simulink model "example1Simulink"  (R2023b)
settings: Solver=VariableStepAuto  StartTime=0.0  StopTime=Tsim  RelTol=1e-3
values from neighbouring files (symbols this model uses):
  C1zA = c2d(C1A,Ts)    [example1Code.m]
  C1zB = c2d(C1B,Ts)    [example1Code.m]
  C1zC = c2d(C1C,Ts)    [example1Code.m]
  finalDisturbance1Value = 0.8    [example1Code.m]
  finalDisturbance2Value = 0.8    [example1Code.m]
  finalReference1Value = 1    [example1Code.m]
  finalReference2Value = 1    [example1Code.m]
  G1z = c2d(G1,Ts)    [example1Code.m]
  initialDisturbance1Value = 0.1    [example1Code.m]
  initialDisturbance2Value = 0.1    [example1Code.m]
  initialReference1Value = 0    [example1Code.m]
  initialReference2Value = 0    [example1Code.m]
  Tref1 = 0    [example1Code.m]
  Tref2 = 15    [example1Code.m]
  Ts = 0.03*sU    (= 0.03)    [example1Code.m]
libraries: cstblocks x24
settings Model: Creator=klysm  LastModifiedBy=klysm

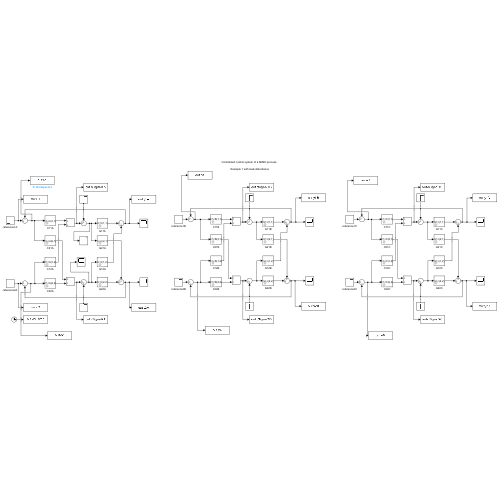
[thumbnail: Simulink's stored preview of the top-level diagram]
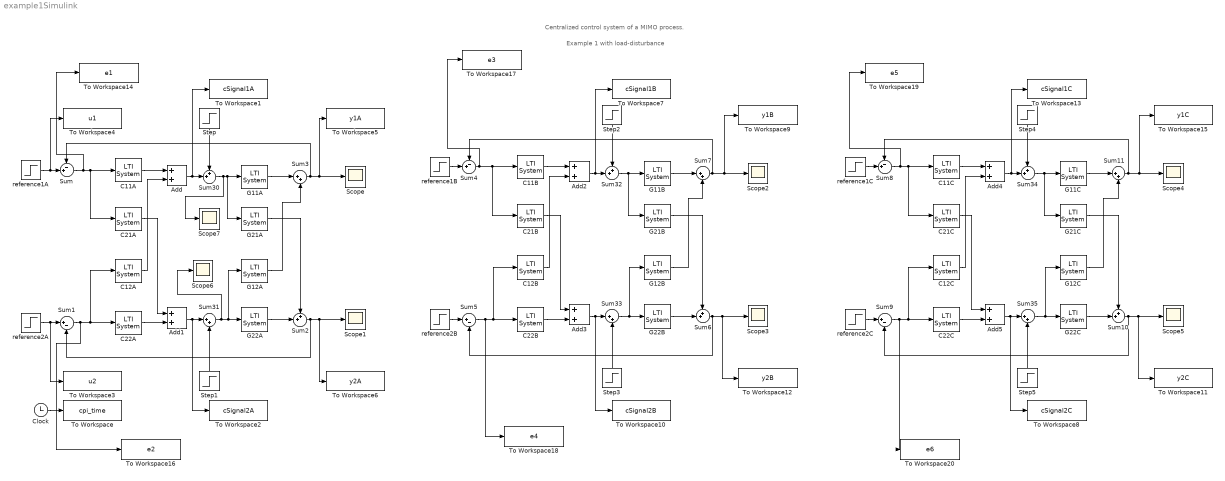
== system example1Simulink ==
  note: Centralized control system of a MIMO process.
  note: Example 1 with load-disturbance
  Add{,1..5} (6 alike) : Sum
  C11A : cstblocks/LTI System  sys=C1zA(1,1)  IC=[]  PadeOrder=0
  C11B : cstblocks/LTI System  sys=C1zB(1,1)  IC=[]  PadeOrder=0
  C11C : cstblocks/LTI System  sys=C1zC(1,1)  IC=[]  PadeOrder=0
  C12A : cstblocks/LTI System  sys=C1zA(1,2)  IC=[]  PadeOrder=0
  C12B : cstblocks/LTI System  sys=C1zB(1,2)  IC=[]  PadeOrder=0
  C12C : cstblocks/LTI System  sys=C1zC(1,2)  IC=[]  PadeOrder=0
  C21A : cstblocks/LTI System  sys=C1zA(2,1)  IC=[]  PadeOrder=0
  C21B : cstblocks/LTI System  sys=C1zB(2,1)  IC=[]  PadeOrder=0
  C21C : cstblocks/LTI System  sys=C1zC(2,1)  IC=[]  PadeOrder=0
  C22A : cstblocks/LTI System  sys=C1zA(2,2)  IC=[]  PadeOrder=0
  C22B : cstblocks/LTI System  sys=C1zB(2,2)  IC=[]  PadeOrder=0
  C22C : cstblocks/LTI System  sys=C1zC(2,2)  IC=[]  PadeOrder=0
  Clock : Clock
  G11A : cstblocks/LTI System  sys=G1z(1,1)  IC=[]  PadeOrder=0
  G11B : cstblocks/LTI System  sys=G1z(1,1)  IC=[]  PadeOrder=0
  G11C : cstblocks/LTI System  sys=G1z(1,1)  IC=[]  PadeOrder=0
  G12A : cstblocks/LTI System  sys=G1z(1,2)  IC=[]  PadeOrder=0
  G12B : cstblocks/LTI System  sys=G1z(1,2)  IC=[]  PadeOrder=0
  G12C : cstblocks/LTI System  sys=G1z(1,2)  IC=[]  PadeOrder=0
  G21A : cstblocks/LTI System  sys=G1z(2,1)  IC=[]  PadeOrder=0
  G21B : cstblocks/LTI System  sys=G1z(2,1)  IC=[]  PadeOrder=0
  G21C : cstblocks/LTI System  sys=G1z(2,1)  IC=[]  PadeOrder=0
  G22A : cstblocks/LTI System  sys=G1z(2,2)  IC=[]  PadeOrder=0
  G22B : cstblocks/LTI System  sys=G1z(2,2)  IC=[]  PadeOrder=0
  G22C : cstblocks/LTI System  sys=G1z(2,2)  IC=[]  PadeOrder=0
  Scope{,1..7} (8 alike) : Scope
  Step : Step  Time=Tref1  Before=initialDisturbance1Value  After=finalDisturbance1Value  SampleTime=Ts
  Step1 : Step  Time=Tref2  Before=initialDisturbance2Value  After=finalDisturbance2Value  SampleTime=Ts
  Step2 : Step  Time=Tref1  Before=initialDisturbance1Value  After=finalDisturbance1Value  SampleTime=Ts
  Step3 : Step  Time=Tref2  Before=initialDisturbance2Value  After=finalDisturbance2Value  SampleTime=Ts
  Step4 : Step  Time=Tref1  Before=initialDisturbance1Value  After=finalDisturbance1Value  SampleTime=Ts
  Step5 : Step  Time=Tref2  Before=initialDisturbance2Value  After=finalDisturbance2Value  SampleTime=Ts
  Sum : Sum  Inputs=-+|
  Sum1 : Sum  Inputs=|+-
  Sum{2,6,10,30,32,34} (6 alike) : Sum  Inputs=++|
  Sum{3,7,11,31,33,35} (6 alike) : Sum  Inputs=|++
  Sum4 : Sum  Inputs=-+|
  Sum5 : Sum  Inputs=|+-
  Sum8 : Sum  Inputs=-+|
  Sum9 : Sum  Inputs=|+-
  To Workspace : ToWorkspace  VariableName=cpi_time  SampleTime=Ts
  To Workspace1 : ToWorkspace  VariableName=cSignal1A  SampleTime=Ts
  To Workspace10 : ToWorkspace  VariableName=cSignal2B  SampleTime=Ts
  To Workspace11 : ToWorkspace  VariableName=y2C  SampleTime=Ts
  To Workspace12 : ToWorkspace  VariableName=y2B  SampleTime=Ts
  To Workspace13 : ToWorkspace  VariableName=cSignal1C  SampleTime=Ts
  To Workspace14 : ToWorkspace  VariableName=e1  SampleTime=Ts
  To Workspace15 : ToWorkspace  VariableName=y1C  SampleTime=Ts
  To Workspace16 : ToWorkspace  VariableName=e2  SampleTime=Ts
  To Workspace17 : ToWorkspace  VariableName=e3  SampleTime=Ts
  To Workspace18 : ToWorkspace  VariableName=e4  SampleTime=Ts
  To Workspace19 : ToWorkspace  VariableName=e5  SampleTime=Ts
  To Workspace2 : ToWorkspace  VariableName=cSignal2A  SampleTime=Ts
  To Workspace20 : ToWorkspace  VariableName=e6  SampleTime=Ts
  To Workspace3 : ToWorkspace  VariableName=u2  SampleTime=Ts
  To Workspace4 : ToWorkspace  VariableName=u1  SampleTime=Ts
  To Workspace5 : ToWorkspace  VariableName=y1A  SampleTime=-1
  To Workspace6 : ToWorkspace  VariableName=y2A  SampleTime=-1
  To Workspace7 : ToWorkspace  VariableName=cSignal1B  SampleTime=Ts
  To Workspace8 : ToWorkspace  VariableName=cSignal2C  SampleTime=Ts
  To Workspace9 : ToWorkspace  VariableName=y1B  SampleTime=Ts
  reference1A : Step  Time=Tref1  Before=initialReference1Value  After=finalReference1Value  SampleTime=Ts
  reference1B : Step  Time=Tref1  Before=initialReference1Value  After=finalReference1Value  SampleTime=Ts
  reference1C : Step  Time=Tref1  Before=initialReference1Value  After=finalReference1Value  SampleTime=Ts
  reference2A : Step  Time=Tref2  Before=initialReference2Value  After=finalReference2Value  SampleTime=Ts
  reference2B : Step  Time=Tref2  Before=initialReference2Value  After=finalReference2Value  SampleTime=Ts
  reference2C : Step  Time=Tref2  Before=initialReference2Value  After=finalReference2Value  SampleTime=Ts
  wires:
  Step4/1 -> Sum34/1
  Sum11/1 -> Sum8/1, To Workspace15/1, Scope4/1
  Add2/1 -> To Workspace7/1, Sum32/2
  C22A/1 -> Add1/2
  C11A/1 -> Add/1
  Step2/1 -> Sum32/1
  Sum35/1 -> G12C/1, G22C/1
  Step/1 -> Sum30/1
  Step5/1 -> Sum35/2
  G12C/1 -> Sum11/2
  G22C/1 -> Sum10/2
  Sum10/1 -> Sum9/2, To Workspace11/1, Scope5/1
  Add5/1 -> To Workspace8/1, Sum35/1
  Sum1/1 -> To Workspace16/1, C12A/1, C22A/1
  reference2A/1 -> To Workspace3/1, Sum1/1
  C21B/1 -> Add3/1
  C11B/1 -> Add2/1
  Add3/1 -> To Workspace10/1, Sum33/1
  Step1/1 -> Sum31/2
  reference1B/1 -> Sum4/2
  Add/1 -> To Workspace1/1, Sum30/2
  Sum30/1 -> Scope7/1, G21A/1, G11A/1
  Add1/1 -> To Workspace2/1, Sum31/1
  reference1C/1 -> Sum8/2
  C12B/1 -> Add2/2
  G12A/1 -> Sum3/2
  C12A/1 -> Add/2
  reference1A/1 -> To Workspace4/1, Sum/2
  C11C/1 -> Add4/1
  Step3/1 -> Sum33/2
  G11C/1 -> Sum11/1
  Sum/1 -> To Workspace14/1, C21A/1, C11A/1
  Sum8/1 -> To Workspace19/1, C21C/1, C11C/1
  C22B/1 -> Add3/2
  Clock/1 -> To Workspace/1
  Sum7/1 -> Sum4/1, To Workspace9/1, Scope2/1
  Sum34/1 -> G21C/1, G11C/1
  G21B/1 -> Sum6/1
  C21C/1 -> Add5/1
  Sum4/1 -> To Workspace17/1, C21B/1, C11B/1
  C21A/1 -> Add1/1
  Add4/1 -> To Workspace13/1, Sum34/2
  Sum3/1 -> Sum/1, To Workspace5/1, Scope/1
  G21C/1 -> Sum10/1
  G21A/1 -> Sum2/1
  reference2C/1 -> Sum9/1
  G12B/1 -> Sum7/2
  Sum33/1 -> G12B/1, G22B/1
  G22A/1 -> Sum2/2
  C22C/1 -> Add5/2
  Sum32/1 -> G21B/1, G11B/1
  Sum6/1 -> Sum5/2, To Workspace12/1, Scope3/1
  Sum5/1 -> To Workspace18/1, C12B/1, C22B/1
  reference2B/1 -> Sum5/1
  G11B/1 -> Sum7/1
  Sum2/1 -> Sum1/2, To Workspace6/1, Scope1/1
  G22B/1 -> Sum6/2
  C12C/1 -> Add4/2
  Sum31/1 -> Scope6/1, G12A/1, G22A/1
  G11A/1 -> Sum3/1
  Sum9/1 -> To Workspace20/1, C12C/1, C22C/1
